simulink model "model"  (R2017a)
settings: Solver=VariableStepAuto  StartTime=0.0  StopTime=10.0  RelTol=1e-3
values from neighbouring files (symbols this model uses):
  Ad = 0.606534330298    [sysd.mat]
  Bd = [-0.0242754206752 -0.00855612972972]    [sysd.mat]
  Cd = [0.128107607141 0.111213837289]    [sysd.mat]
  Dd = [-0.0321285947629  0.0590346867599; -0.035674975325  0.0556784277831]    [sysd.mat]
  Ts = 6.438500000000000    (= 6.4385)    [Initialization.m]    (also in sysd.mat)
undefined symbols (not defined in the file or in its folder): Ed, Kd
libraries: simulink x2
settings Model: Creator=nvink  LastModifiedBy=nvink

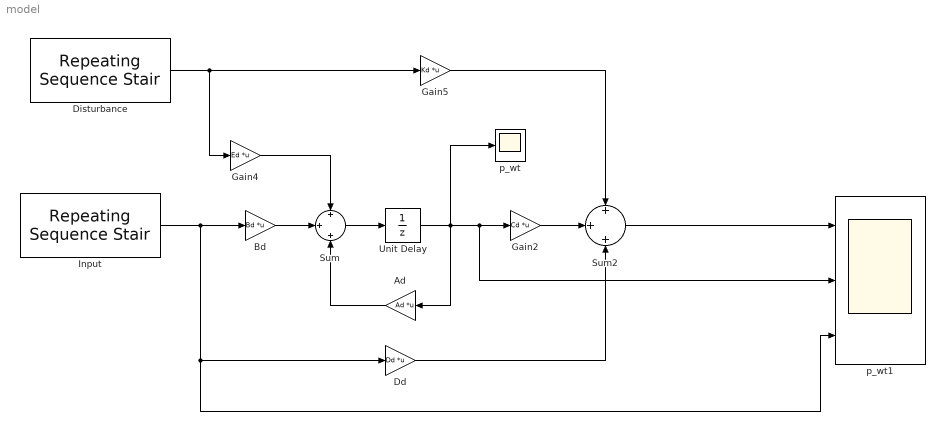
== system model ==
  Ad : Gain  Gain=Ad  Multiplication=Matrix(K*u)
      mask Display:
      | %color('cyan')
      | color('magenta')
      | disp('{\bf\fontsize{14}Ad}', 'texmode','on');
      | %disp('Ad')
  Bd : Gain  Gain=Bd  Multiplication=Matrix(K*u)
      mask Display:
      | %color('cyan')
      | color('magenta')
      | disp('{\bf\fontsize{14}Bd}', 'texmode','on');
      | %disp('Bd')
  Dd : Gain  Gain=Dd  Multiplication=Matrix(K*u)
      mask Display:
      | %color('cyan')
      | color('magenta')
      | disp('{\bf\fontsize{14}Dd}', 'texmode','on');
      | %disp('Dd')
  Disturbance : simulink/Sources/Repeating Sequence Stair  OutValues=constant_dist  tsamp=3600  OutMin=[]  OutMax=[]  OutDataTypeStr=double  OutputDataTypeScalingMode=double  OutDataType=fixdt(0,8)  ConRadixGroup=Best Precision: Vector-wise  OutScaling=2^-12
  Gain2 : Gain  Gain=Cd  Multiplication=Matrix(K*u)
      mask Display:
      | %color('cyan')
      | color('magenta')
      | disp('{\bf\fontsize{14}Cd}', 'texmode','on');
      | %disp('Cd')
  Gain4 : Gain  Gain=Ed  Multiplication=Matrix(K*u)
      mask Display:
      | %color('cyan')
      | color('magenta')
      | disp('{\bf\fontsize{14}Ed}', 'texmode','on');
      | %disp('Ed')
  Gain5 : Gain  Gain=Kd  Multiplication=Matrix(K*u)
      mask Display:
      | %color('cyan')
      | color('magenta')
      | disp('{\bf\fontsize{14}Kd}', 'texmode','on');
      | %disp('Kd')
  Input : simulink/Sources/Repeating Sequence Stair  OutValues=ones(100,1)  tsamp=3600  OutMin=[]  OutMax=[]  OutDataTypeStr=double  OutputDataTypeScalingMode=double  OutDataType=fixdt(0,8)  ConRadixGroup=Best Precision: Vector-wise  OutScaling=2^-12
  Sum : Sum  Inputs=+|+|+
  Sum2 : Sum  Inputs=+|+|+
  Unit Delay : UnitDelay  InitialCondition=0.005  SampleTime=Ts
  p_wt : Scope
  p_wt1 : Scope  NumInputPorts=3
  wires:
  Gain5/1 -> Sum2/1
  Dd/1 -> Sum2/3
  Gain2/1 -> Sum2/2
  Gain4/1 -> Sum/1
  Sum2/1 -> p_wt1/1
  Unit Delay/1 -> p_wt/1, p_wt1/2, Gain2/1, Ad/1
  Disturbance/1 -> Gain4/1, Gain5/1
  Bd/1 -> Sum/2
  Input/1 -> p_wt1/3, Dd/1, Bd/1
  Ad/1 -> Sum/3
  Sum/1 -> Unit Delay/1
